simulink model "TST_CrCtl_Governor"  (R2016b)
settings: Solver=FixedStepDiscrete  StartTime=0.0  StopTime=simTime  FixedStep=sampleTime  RelTol=1e-3
values from neighbouring files (symbols this model uses):
  testCase = 1    [initTST_CrCtl_Governor_001.m]    (also in initTST_CrCtl_Governor_002.m = 2; initTST_CrCtl_Governor_003.m = 3; initTST_CrCtl_Governor_004.m = 4; initTST_CrCtl_Governor_005.m = 5)
libraries: simulink x144, UnitTest_Lib x110
(part 3 of 7)

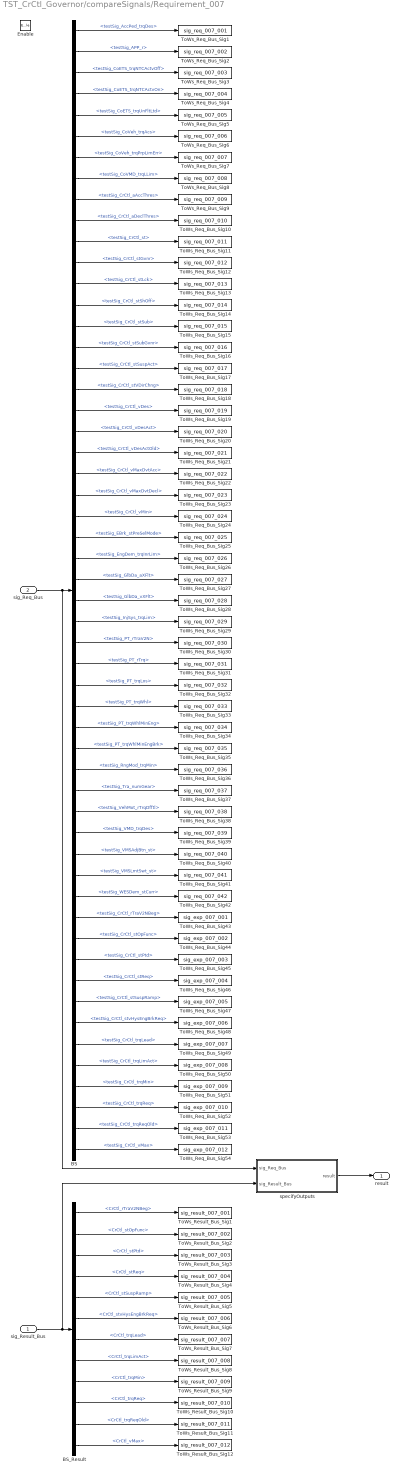
== system TST_CrCtl_Governor/compareSignals/Requirement_007 ==
  sig_Result_Bus : Inport
  sig_Req_Bus : Inport  Port=2
  Enable : EnablePort
  BS : BusSelector  OutputSignals=testSig_AccPed_trqDes,testSig_APP_r,testSig_CoETS_trqNTCActvOff,testSig_CoETS_trqNTCActvOn,testSig_CoETS_trqUnFltLtd,testSig_CoVeh_trqAcs,testSig_CoVeh_trqPrpLimErr,testSig_CoVMD_trqLLim,testSig_CrCtl_aAccThres,testSig_CrCtl_aDeclThres,testSig_CrCtl_st,testSig_CrCtl_stGvnr,testSig_CrCtl_stLck,testSig_CrCtl_stShOff,testSig_CrCtl_stSub,testSig_CrCtl_stSubGvnr,testSig_CrCtl_stSuspAct,testSig_CrCtl_stVDirChng,testSig_CrCtl_vDes,testSig_CrCtl_vDesAct,testSig_CrCtl_vDesActOld,testSig_CrCtl_vMaxDvtAcc,testSig_CrCtl_vMaxDvtDecl,testSig_CrCtl_vMin,testSig_EBrk_stPreSelMode,testSig_EngDem_trqInrLim,testSig_GlbDa_aXFlt,testSig_GlbDa_vXFlt,testSig_InjSys_trqLim,testSig_PT_rTraV2N,testSig_PT_rTrq,testSig_PT_trqLos,testSig_PT_trqWhl,testSig_PT_trqWhlMinEng,testSig_PT_trqWhlMinEngBrk,testSig_RngMod_trqMin,testSig_Tra_numGear,testSig_VehMot_rTrqDfftl,testSig_VMD_trqDes,testSig_VMSAdjBtn_st,testSig_VMSLmtSwt_st,testSig_WESDem_stCurr,testSig_CrCtl_rTraV2NBeg,testSig_CrCtl_stOpFunc,testSig_CrCtl_stPtd,testSig_CrCtl_stReq,testSig_CrCtl_stSuspRamp,testSig_CrCtl_stvHysEngBrkReq,testSig_CrCtl_trqLead,testSig_CrCtl_trqLimAct,testSig_CrCtl_trqMin,testSig_CrCtl_trqReq,testSig_CrCtl_trqReqOld,testSig_CrCtl_vMax
  BS_Result : BusSelector  OutputSignals=CrCtl_rTraV2NBeg,CrCtl_stOpFunc,CrCtl_stPtd,CrCtl_stReq,CrCtl_stSuspRamp,CrCtl_stvHysEngBrkReq,CrCtl_trqLead,CrCtl_trqLimAct,CrCtl_trqMin,CrCtl_trqReq,CrCtl_trqReqOld,CrCtl_vMax
  ToWs_Req_Bus_Sig1 : ToWorkspace  VariableName=sig_req_007_001  SaveFormat=Structure With Time
  ToWs_Req_Bus_Sig10 : ToWorkspace  VariableName=sig_req_007_010  SaveFormat=Structure With Time
  ToWs_Req_Bus_Sig11 : ToWorkspace  VariableName=sig_req_007_011  SaveFormat=Structure With Time
  ToWs_Req_Bus_Sig12 : ToWorkspace  VariableName=sig_req_007_012  SaveFormat=Structure With Time
  ToWs_Req_Bus_Sig13 : ToWorkspace  VariableName=sig_req_007_013  SaveFormat=Structure With Time
  ToWs_Req_Bus_Sig14 : ToWorkspace  VariableName=sig_req_007_014  SaveFormat=Structure With Time
  ToWs_Req_Bus_Sig15 : ToWorkspace  VariableName=sig_req_007_015  SaveFormat=Structure With Time
  ToWs_Req_Bus_Sig16 : ToWorkspace  VariableName=sig_req_007_016  SaveFormat=Structure With Time
  ToWs_Req_Bus_Sig17 : ToWorkspace  VariableName=sig_req_007_017  SaveFormat=Structure With Time
  ToWs_Req_Bus_Sig18 : ToWorkspace  VariableName=sig_req_007_018  SaveFormat=Structure With Time
  ToWs_Req_Bus_Sig19 : ToWorkspace  VariableName=sig_req_007_019  SaveFormat=Structure With Time
  ToWs_Req_Bus_Sig2 : ToWorkspace  VariableName=sig_req_007_002  SaveFormat=Structure With Time
  ToWs_Req_Bus_Sig20 : ToWorkspace  VariableName=sig_req_007_020  SaveFormat=Structure With Time
  ToWs_Req_Bus_Sig21 : ToWorkspace  VariableName=sig_req_007_021  SaveFormat=Structure With Time
  ToWs_Req_Bus_Sig22 : ToWorkspace  VariableName=sig_req_007_022  SaveFormat=Structure With Time
  ToWs_Req_Bus_Sig23 : ToWorkspace  VariableName=sig_req_007_023  SaveFormat=Structure With Time
  ToWs_Req_Bus_Sig24 : ToWorkspace  VariableName=sig_req_007_024  SaveFormat=Structure With Time
  ToWs_Req_Bus_Sig25 : ToWorkspace  VariableName=sig_req_007_025  SaveFormat=Structure With Time
  ToWs_Req_Bus_Sig26 : ToWorkspace  VariableName=sig_req_007_026  SaveFormat=Structure With Time
  ToWs_Req_Bus_Sig27 : ToWorkspace  VariableName=sig_req_007_027  SaveFormat=Structure With Time
  ToWs_Req_Bus_Sig28 : ToWorkspace  VariableName=sig_req_007_028  SaveFormat=Structure With Time
  ToWs_Req_Bus_Sig29 : ToWorkspace  VariableName=sig_req_007_029  SaveFormat=Structure With Time
  ToWs_Req_Bus_Sig3 : ToWorkspace  VariableName=sig_req_007_003  SaveFormat=Structure With Time
  ToWs_Req_Bus_Sig30 : ToWorkspace  VariableName=sig_req_007_030  SaveFormat=Structure With Time
  ToWs_Req_Bus_Sig31 : ToWorkspace  VariableName=sig_req_007_031  SaveFormat=Structure With Time
  ToWs_Req_Bus_Sig32 : ToWorkspace  VariableName=sig_req_007_032  SaveFormat=Structure With Time
  ToWs_Req_Bus_Sig33 : ToWorkspace  VariableName=sig_req_007_033  SaveFormat=Structure With Time
  ToWs_Req_Bus_Sig34 : ToWorkspace  VariableName=sig_req_007_034  SaveFormat=Structure With Time
  ToWs_Req_Bus_Sig35 : ToWorkspace  VariableName=sig_req_007_035  SaveFormat=Structure With Time
  ToWs_Req_Bus_Sig36 : ToWorkspace  VariableName=sig_req_007_036  SaveFormat=Structure With Time
  ToWs_Req_Bus_Sig37 : ToWorkspace  VariableName=sig_req_007_037  SaveFormat=Structure With Time
  ToWs_Req_Bus_Sig38 : ToWorkspace  VariableName=sig_req_007_038  SaveFormat=Structure With Time
  ToWs_Req_Bus_Sig39 : ToWorkspace  VariableName=sig_req_007_039  SaveFormat=Structure With Time
  ToWs_Req_Bus_Sig4 : ToWorkspace  VariableName=sig_req_007_004  SaveFormat=Structure With Time
  ToWs_Req_Bus_Sig40 : ToWorkspace  VariableName=sig_req_007_040  SaveFormat=Structure With Time
  ToWs_Req_Bus_Sig41 : ToWorkspace  VariableName=sig_req_007_041  SaveFormat=Structure With Time
  ToWs_Req_Bus_Sig42 : ToWorkspace  VariableName=sig_req_007_042  SaveFormat=Structure With Time
  ToWs_Req_Bus_Sig43 : ToWorkspace  VariableName=sig_exp_007_001  SaveFormat=Structure With Time
  ToWs_Req_Bus_Sig44 : ToWorkspace  VariableName=sig_exp_007_002  SaveFormat=Structure With Time
  ToWs_Req_Bus_Sig45 : ToWorkspace  VariableName=sig_exp_007_003  SaveFormat=Structure With Time
  ToWs_Req_Bus_Sig46 : ToWorkspace  VariableName=sig_exp_007_004  SaveFormat=Structure With Time
  ToWs_Req_Bus_Sig47 : ToWorkspace  VariableName=sig_exp_007_005  SaveFormat=Structure With Time
  ToWs_Req_Bus_Sig48 : ToWorkspace  VariableName=sig_exp_007_006  SaveFormat=Structure With Time
  ToWs_Req_Bus_Sig49 : ToWorkspace  VariableName=sig_exp_007_007  SaveFormat=Structure With Time
  ToWs_Req_Bus_Sig5 : ToWorkspace  VariableName=sig_req_007_005  SaveFormat=Structure With Time
  ToWs_Req_Bus_Sig50 : ToWorkspace  VariableName=sig_exp_007_008  SaveFormat=Structure With Time
  ToWs_Req_Bus_Sig51 : ToWorkspace  VariableName=sig_exp_007_009  SaveFormat=Structure With Time
  ToWs_Req_Bus_Sig52 : ToWorkspace  VariableName=sig_exp_007_010  SaveFormat=Structure With Time
  ToWs_Req_Bus_Sig53 : ToWorkspace  VariableName=sig_exp_007_011  SaveFormat=Structure With Time
  ToWs_Req_Bus_Sig54 : ToWorkspace  VariableName=sig_exp_007_012  SaveFormat=Structure With Time
  ToWs_Req_Bus_Sig6 : ToWorkspace  VariableName=sig_req_007_006  SaveFormat=Structure With Time
  ToWs_Req_Bus_Sig7 : ToWorkspace  VariableName=sig_req_007_007  SaveFormat=Structure With Time
  ToWs_Req_Bus_Sig8 : ToWorkspace  VariableName=sig_req_007_008  SaveFormat=Structure With Time
  ToWs_Req_Bus_Sig9 : ToWorkspace  VariableName=sig_req_007_009  SaveFormat=Structure With Time
  ToWs_Result_Bus_Sig1 : ToWorkspace  VariableName=sig_result_007_001  SaveFormat=Structure With Time
  ToWs_Result_Bus_Sig10 : ToWorkspace  VariableName=sig_result_007_010  SaveFormat=Structure With Time
  ToWs_Result_Bus_Sig11 : ToWorkspace  VariableName=sig_result_007_011  SaveFormat=Structure With Time
  ToWs_Result_Bus_Sig12 : ToWorkspace  VariableName=sig_result_007_012  SaveFormat=Structure With Time
  ToWs_Result_Bus_Sig2 : ToWorkspace  VariableName=sig_result_007_002  SaveFormat=Structure With Time
  ToWs_Result_Bus_Sig3 : ToWorkspace  VariableName=sig_result_007_003  SaveFormat=Structure With Time
  ToWs_Result_Bus_Sig4 : ToWorkspace  VariableName=sig_result_007_004  SaveFormat=Structure With Time
  ToWs_Result_Bus_Sig5 : ToWorkspace  VariableName=sig_result_007_005  SaveFormat=Structure With Time
  ToWs_Result_Bus_Sig6 : ToWorkspace  VariableName=sig_result_007_006  SaveFormat=Structure With Time
  ToWs_Result_Bus_Sig7 : ToWorkspace  VariableName=sig_result_007_007  SaveFormat=Structure With Time
  ToWs_Result_Bus_Sig8 : ToWorkspace  VariableName=sig_result_007_008  SaveFormat=Structure With Time
  ToWs_Result_Bus_Sig9 : ToWorkspace  VariableName=sig_result_007_009  SaveFormat=Structure With Time
  specifyOutputs : Subsystem
  result : Outport
  wires:
  sig_Req_Bus/1 -> BS/1, specifyOutputs/1(sig_Req_Bus)
  BS/1 -> ToWs_Req_Bus_Sig1/1  "<testSig_AccPed_trqDes>"
  BS/2 -> ToWs_Req_Bus_Sig2/1  "<testSig_APP_r>"
  BS/3 -> ToWs_Req_Bus_Sig3/1  "<testSig_CoETS_trqNTCActvOff>"
  BS/4 -> ToWs_Req_Bus_Sig4/1  "<testSig_CoETS_trqNTCActvOn>"
  BS/5 -> ToWs_Req_Bus_Sig5/1  "<testSig_CoETS_trqUnFltLtd>"
  BS/6 -> ToWs_Req_Bus_Sig6/1  "<testSig_CoVeh_trqAcs>"
  BS/7 -> ToWs_Req_Bus_Sig7/1  "<testSig_CoVeh_trqPrpLimErr>"
  BS/8 -> ToWs_Req_Bus_Sig8/1  "<testSig_CoVMD_trqLLim>"
  BS/9 -> ToWs_Req_Bus_Sig9/1  "<testSig_CrCtl_aAccThres>"
  BS/10 -> ToWs_Req_Bus_Sig10/1  "<testSig_CrCtl_aDeclThres>"
  BS/11 -> ToWs_Req_Bus_Sig11/1  "<testSig_CrCtl_st>"
  BS/12 -> ToWs_Req_Bus_Sig12/1  "<testSig_CrCtl_stGvnr>"
  BS/13 -> ToWs_Req_Bus_Sig13/1  "<testSig_CrCtl_stLck>"
  BS/14 -> ToWs_Req_Bus_Sig14/1  "<testSig_CrCtl_stShOff>"
  BS/15 -> ToWs_Req_Bus_Sig15/1  "<testSig_CrCtl_stSub>"
  BS/16 -> ToWs_Req_Bus_Sig16/1  "<testSig_CrCtl_stSubGvnr>"
  BS/17 -> ToWs_Req_Bus_Sig17/1  "<testSig_CrCtl_stSuspAct>"
  BS/18 -> ToWs_Req_Bus_Sig18/1  "<testSig_CrCtl_stVDirChng>"
  BS/19 -> ToWs_Req_Bus_Sig19/1  "<testSig_CrCtl_vDes>"
  BS/20 -> ToWs_Req_Bus_Sig20/1  "<testSig_CrCtl_vDesAct>"
  BS/21 -> ToWs_Req_Bus_Sig21/1  "<testSig_CrCtl_vDesActOld>"
  BS/22 -> ToWs_Req_Bus_Sig22/1  "<testSig_CrCtl_vMaxDvtAcc>"
  BS/23 -> ToWs_Req_Bus_Sig23/1  "<testSig_CrCtl_vMaxDvtDecl>"
  BS/24 -> ToWs_Req_Bus_Sig24/1  "<testSig_CrCtl_vMin>"
  BS/25 -> ToWs_Req_Bus_Sig25/1  "<testSig_EBrk_stPreSelMode>"
  BS/26 -> ToWs_Req_Bus_Sig26/1  "<testSig_EngDem_trqInrLim>"
  BS/27 -> ToWs_Req_Bus_Sig27/1  "<testSig_GlbDa_aXFlt>"
  BS/28 -> ToWs_Req_Bus_Sig28/1  "<testSig_GlbDa_vXFlt>"
  BS/29 -> ToWs_Req_Bus_Sig29/1  "<testSig_InjSys_trqLim>"
  BS/30 -> ToWs_Req_Bus_Sig30/1  "<testSig_PT_rTraV2N>"
  BS/31 -> ToWs_Req_Bus_Sig31/1  "<testSig_PT_rTrq>"
  BS/32 -> ToWs_Req_Bus_Sig32/1  "<testSig_PT_trqLos>"
  BS/33 -> ToWs_Req_Bus_Sig33/1  "<testSig_PT_trqWhl>"
  BS/34 -> ToWs_Req_Bus_Sig34/1  "<testSig_PT_trqWhlMinEng>"
  BS/35 -> ToWs_Req_Bus_Sig35/1  "<testSig_PT_trqWhlMinEngBrk>"
  BS/36 -> ToWs_Req_Bus_Sig36/1  "<testSig_RngMod_trqMin>"
  BS/37 -> ToWs_Req_Bus_Sig37/1  "<testSig_Tra_numGear>"
  BS/38 -> ToWs_Req_Bus_Sig38/1  "<testSig_VehMot_rTrqDfftl>"
  BS/39 -> ToWs_Req_Bus_Sig39/1  "<testSig_VMD_trqDes>"
  BS/40 -> ToWs_Req_Bus_Sig40/1  "<testSig_VMSAdjBtn_st>"
  BS/41 -> ToWs_Req_Bus_Sig41/1  "<testSig_VMSLmtSwt_st>"
  BS/42 -> ToWs_Req_Bus_Sig42/1  "<testSig_WESDem_stCurr>"
  BS/43 -> ToWs_Req_Bus_Sig43/1  "<testSig_CrCtl_rTraV2NBeg>"
  BS/44 -> ToWs_Req_Bus_Sig44/1  "<testSig_CrCtl_stOpFunc>"
  BS/45 -> ToWs_Req_Bus_Sig45/1  "<testSig_CrCtl_stPtd>"
  BS/46 -> ToWs_Req_Bus_Sig46/1  "<testSig_CrCtl_stReq>"
  BS/47 -> ToWs_Req_Bus_Sig47/1  "<testSig_CrCtl_stSuspRamp>"
  BS/48 -> ToWs_Req_Bus_Sig48/1  "<testSig_CrCtl_stvHysEngBrkReq>"
  BS/49 -> ToWs_Req_Bus_Sig49/1  "<testSig_CrCtl_trqLead>"
  BS/50 -> ToWs_Req_Bus_Sig50/1  "<testSig_CrCtl_trqLimAct>"
  BS/51 -> ToWs_Req_Bus_Sig51/1  "<testSig_CrCtl_trqMin>"
  BS/52 -> ToWs_Req_Bus_Sig52/1  "<testSig_CrCtl_trqReq>"
  BS/53 -> ToWs_Req_Bus_Sig53/1  "<testSig_CrCtl_trqReqOld>"
  BS/54 -> ToWs_Req_Bus_Sig54/1  "<testSig_CrCtl_vMax>"
  sig_Result_Bus/1 -> BS_Result/1, specifyOutputs/2(sig_Result_Bus)
  BS_Result/1 -> ToWs_Result_Bus_Sig1/1  "<CrCtl_rTraV2NBeg>"
  BS_Result/2 -> ToWs_Result_Bus_Sig2/1  "<CrCtl_stOpFunc>"
  BS_Result/3 -> ToWs_Result_Bus_Sig3/1  "<CrCtl_stPtd>"
  BS_Result/4 -> ToWs_Result_Bus_Sig4/1  "<CrCtl_stReq>"
  BS_Result/5 -> ToWs_Result_Bus_Sig5/1  "<CrCtl_stSuspRamp>"
  BS_Result/6 -> ToWs_Result_Bus_Sig6/1  "<CrCtl_stvHysEngBrkReq>"
  BS_Result/7 -> ToWs_Result_Bus_Sig7/1  "<CrCtl_trqLead>"
  BS_Result/8 -> ToWs_Result_Bus_Sig8/1  "<CrCtl_trqLimAct>"
  BS_Result/9 -> ToWs_Result_Bus_Sig9/1  "<CrCtl_trqMin>"
  BS_Result/10 -> ToWs_Result_Bus_Sig10/1  "<CrCtl_trqReq>"
  BS_Result/11 -> ToWs_Result_Bus_Sig11/1  "<CrCtl_trqReqOld>"
  BS_Result/12 -> ToWs_Result_Bus_Sig12/1  "<CrCtl_vMax>"
  specifyOutputs/1(result) -> result/1

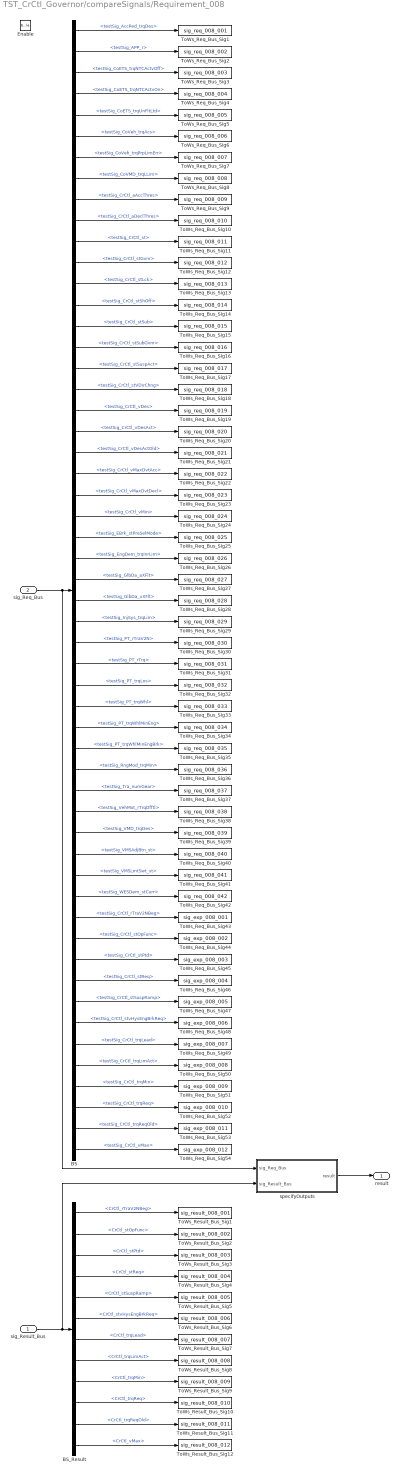
== system TST_CrCtl_Governor/compareSignals/Requirement_008 ==
  sig_Result_Bus : Inport
  sig_Req_Bus : Inport  Port=2
  Enable : EnablePort
  BS : BusSelector  OutputSignals=testSig_AccPed_trqDes,testSig_APP_r,testSig_CoETS_trqNTCActvOff,testSig_CoETS_trqNTCActvOn,testSig_CoETS_trqUnFltLtd,testSig_CoVeh_trqAcs,testSig_CoVeh_trqPrpLimErr,testSig_CoVMD_trqLLim,testSig_CrCtl_aAccThres,testSig_CrCtl_aDeclThres,testSig_CrCtl_st,testSig_CrCtl_stGvnr,testSig_CrCtl_stLck,testSig_CrCtl_stShOff,testSig_CrCtl_stSub,testSig_CrCtl_stSubGvnr,testSig_CrCtl_stSuspAct,testSig_CrCtl_stVDirChng,testSig_CrCtl_vDes,testSig_CrCtl_vDesAct,testSig_CrCtl_vDesActOld,testSig_CrCtl_vMaxDvtAcc,testSig_CrCtl_vMaxDvtDecl,testSig_CrCtl_vMin,testSig_EBrk_stPreSelMode,testSig_EngDem_trqInrLim,testSig_GlbDa_aXFlt,testSig_GlbDa_vXFlt,testSig_InjSys_trqLim,testSig_PT_rTraV2N,testSig_PT_rTrq,testSig_PT_trqLos,testSig_PT_trqWhl,testSig_PT_trqWhlMinEng,testSig_PT_trqWhlMinEngBrk,testSig_RngMod_trqMin,testSig_Tra_numGear,testSig_VehMot_rTrqDfftl,testSig_VMD_trqDes,testSig_VMSAdjBtn_st,testSig_VMSLmtSwt_st,testSig_WESDem_stCurr,testSig_CrCtl_rTraV2NBeg,testSig_CrCtl_stOpFunc,testSig_CrCtl_stPtd,testSig_CrCtl_stReq,testSig_CrCtl_stSuspRamp,testSig_CrCtl_stvHysEngBrkReq,testSig_CrCtl_trqLead,testSig_CrCtl_trqLimAct,testSig_CrCtl_trqMin,testSig_CrCtl_trqReq,testSig_CrCtl_trqReqOld,testSig_CrCtl_vMax
  BS_Result : BusSelector  OutputSignals=CrCtl_rTraV2NBeg,CrCtl_stOpFunc,CrCtl_stPtd,CrCtl_stReq,CrCtl_stSuspRamp,CrCtl_stvHysEngBrkReq,CrCtl_trqLead,CrCtl_trqLimAct,CrCtl_trqMin,CrCtl_trqReq,CrCtl_trqReqOld,CrCtl_vMax
  ToWs_Req_Bus_Sig1 : ToWorkspace  VariableName=sig_req_008_001  SaveFormat=Structure With Time
  ToWs_Req_Bus_Sig10 : ToWorkspace  VariableName=sig_req_008_010  SaveFormat=Structure With Time
  ToWs_Req_Bus_Sig11 : ToWorkspace  VariableName=sig_req_008_011  SaveFormat=Structure With Time
  ToWs_Req_Bus_Sig12 : ToWorkspace  VariableName=sig_req_008_012  SaveFormat=Structure With Time
  ToWs_Req_Bus_Sig13 : ToWorkspace  VariableName=sig_req_008_013  SaveFormat=Structure With Time
  ToWs_Req_Bus_Sig14 : ToWorkspace  VariableName=sig_req_008_014  SaveFormat=Structure With Time
  ToWs_Req_Bus_Sig15 : ToWorkspace  VariableName=sig_req_008_015  SaveFormat=Structure With Time
  ToWs_Req_Bus_Sig16 : ToWorkspace  VariableName=sig_req_008_016  SaveFormat=Structure With Time
  ToWs_Req_Bus_Sig17 : ToWorkspace  VariableName=sig_req_008_017  SaveFormat=Structure With Time
  ToWs_Req_Bus_Sig18 : ToWorkspace  VariableName=sig_req_008_018  SaveFormat=Structure With Time
  ToWs_Req_Bus_Sig19 : ToWorkspace  VariableName=sig_req_008_019  SaveFormat=Structure With Time
  ToWs_Req_Bus_Sig2 : ToWorkspace  VariableName=sig_req_008_002  SaveFormat=Structure With Time
  ToWs_Req_Bus_Sig20 : ToWorkspace  VariableName=sig_req_008_020  SaveFormat=Structure With Time
  ToWs_Req_Bus_Sig21 : ToWorkspace  VariableName=sig_req_008_021  SaveFormat=Structure With Time
  ToWs_Req_Bus_Sig22 : ToWorkspace  VariableName=sig_req_008_022  SaveFormat=Structure With Time
  ToWs_Req_Bus_Sig23 : ToWorkspace  VariableName=sig_req_008_023  SaveFormat=Structure With Time
  ToWs_Req_Bus_Sig24 : ToWorkspace  VariableName=sig_req_008_024  SaveFormat=Structure With Time
  ToWs_Req_Bus_Sig25 : ToWorkspace  VariableName=sig_req_008_025  SaveFormat=Structure With Time
  ToWs_Req_Bus_Sig26 : ToWorkspace  VariableName=sig_req_008_026  SaveFormat=Structure With Time
  ToWs_Req_Bus_Sig27 : ToWorkspace  VariableName=sig_req_008_027  SaveFormat=Structure With Time
  ToWs_Req_Bus_Sig28 : ToWorkspace  VariableName=sig_req_008_028  SaveFormat=Structure With Time
  ToWs_Req_Bus_Sig29 : ToWorkspace  VariableName=sig_req_008_029  SaveFormat=Structure With Time
  ToWs_Req_Bus_Sig3 : ToWorkspace  VariableName=sig_req_008_003  SaveFormat=Structure With Time
  ToWs_Req_Bus_Sig30 : ToWorkspace  VariableName=sig_req_008_030  SaveFormat=Structure With Time
  ToWs_Req_Bus_Sig31 : ToWorkspace  VariableName=sig_req_008_031  SaveFormat=Structure With Time
  ToWs_Req_Bus_Sig32 : ToWorkspace  VariableName=sig_req_008_032  SaveFormat=Structure With Time
  ToWs_Req_Bus_Sig33 : ToWorkspace  VariableName=sig_req_008_033  SaveFormat=Structure With Time
  ToWs_Req_Bus_Sig34 : ToWorkspace  VariableName=sig_req_008_034  SaveFormat=Structure With Time
  ToWs_Req_Bus_Sig35 : ToWorkspace  VariableName=sig_req_008_035  SaveFormat=Structure With Time
  ToWs_Req_Bus_Sig36 : ToWorkspace  VariableName=sig_req_008_036  SaveFormat=Structure With Time
  ToWs_Req_Bus_Sig37 : ToWorkspace  VariableName=sig_req_008_037  SaveFormat=Structure With Time
  ToWs_Req_Bus_Sig38 : ToWorkspace  VariableName=sig_req_008_038  SaveFormat=Structure With Time
  ToWs_Req_Bus_Sig39 : ToWorkspace  VariableName=sig_req_008_039  SaveFormat=Structure With Time
  ToWs_Req_Bus_Sig4 : ToWorkspace  VariableName=sig_req_008_004  SaveFormat=Structure With Time
  ToWs_Req_Bus_Sig40 : ToWorkspace  VariableName=sig_req_008_040  SaveFormat=Structure With Time
  ToWs_Req_Bus_Sig41 : ToWorkspace  VariableName=sig_req_008_041  SaveFormat=Structure With Time
  ToWs_Req_Bus_Sig42 : ToWorkspace  VariableName=sig_req_008_042  SaveFormat=Structure With Time
  ToWs_Req_Bus_Sig43 : ToWorkspace  VariableName=sig_exp_008_001  SaveFormat=Structure With Time
  ToWs_Req_Bus_Sig44 : ToWorkspace  VariableName=sig_exp_008_002  SaveFormat=Structure With Time
  ToWs_Req_Bus_Sig45 : ToWorkspace  VariableName=sig_exp_008_003  SaveFormat=Structure With Time
  ToWs_Req_Bus_Sig46 : ToWorkspace  VariableName=sig_exp_008_004  SaveFormat=Structure With Time
  ToWs_Req_Bus_Sig47 : ToWorkspace  VariableName=sig_exp_008_005  SaveFormat=Structure With Time
  ToWs_Req_Bus_Sig48 : ToWorkspace  VariableName=sig_exp_008_006  SaveFormat=Structure With Time
  ToWs_Req_Bus_Sig49 : ToWorkspace  VariableName=sig_exp_008_007  SaveFormat=Structure With Time
  ToWs_Req_Bus_Sig5 : ToWorkspace  VariableName=sig_req_008_005  SaveFormat=Structure With Time
  ToWs_Req_Bus_Sig50 : ToWorkspace  VariableName=sig_exp_008_008  SaveFormat=Structure With Time
  ToWs_Req_Bus_Sig51 : ToWorkspace  VariableName=sig_exp_008_009  SaveFormat=Structure With Time
  ToWs_Req_Bus_Sig52 : ToWorkspace  VariableName=sig_exp_008_010  SaveFormat=Structure With Time
  ToWs_Req_Bus_Sig53 : ToWorkspace  VariableName=sig_exp_008_011  SaveFormat=Structure With Time
  ToWs_Req_Bus_Sig54 : ToWorkspace  VariableName=sig_exp_008_012  SaveFormat=Structure With Time
  ToWs_Req_Bus_Sig6 : ToWorkspace  VariableName=sig_req_008_006  SaveFormat=Structure With Time
  ToWs_Req_Bus_Sig7 : ToWorkspace  VariableName=sig_req_008_007  SaveFormat=Structure With Time
  ToWs_Req_Bus_Sig8 : ToWorkspace  VariableName=sig_req_008_008  SaveFormat=Structure With Time
  ToWs_Req_Bus_Sig9 : ToWorkspace  VariableName=sig_req_008_009  SaveFormat=Structure With Time
  ToWs_Result_Bus_Sig1 : ToWorkspace  VariableName=sig_result_008_001  SaveFormat=Structure With Time
  ToWs_Result_Bus_Sig10 : ToWorkspace  VariableName=sig_result_008_010  SaveFormat=Structure With Time
  ToWs_Result_Bus_Sig11 : ToWorkspace  VariableName=sig_result_008_011  SaveFormat=Structure With Time
  ToWs_Result_Bus_Sig12 : ToWorkspace  VariableName=sig_result_008_012  SaveFormat=Structure With Time
  ToWs_Result_Bus_Sig2 : ToWorkspace  VariableName=sig_result_008_002  SaveFormat=Structure With Time
  ToWs_Result_Bus_Sig3 : ToWorkspace  VariableName=sig_result_008_003  SaveFormat=Structure With Time
  ToWs_Result_Bus_Sig4 : ToWorkspace  VariableName=sig_result_008_004  SaveFormat=Structure With Time
  ToWs_Result_Bus_Sig5 : ToWorkspace  VariableName=sig_result_008_005  SaveFormat=Structure With Time
  ToWs_Result_Bus_Sig6 : ToWorkspace  VariableName=sig_result_008_006  SaveFormat=Structure With Time
  ToWs_Result_Bus_Sig7 : ToWorkspace  VariableName=sig_result_008_007  SaveFormat=Structure With Time
  ToWs_Result_Bus_Sig8 : ToWorkspace  VariableName=sig_result_008_008  SaveFormat=Structure With Time
  ToWs_Result_Bus_Sig9 : ToWorkspace  VariableName=sig_result_008_009  SaveFormat=Structure With Time
  specifyOutputs : Subsystem
  result : Outport
  wires:
  sig_Req_Bus/1 -> BS/1, specifyOutputs/1(sig_Req_Bus)
  BS/1 -> ToWs_Req_Bus_Sig1/1  "<testSig_AccPed_trqDes>"
  BS/2 -> ToWs_Req_Bus_Sig2/1  "<testSig_APP_r>"
  BS/3 -> ToWs_Req_Bus_Sig3/1  "<testSig_CoETS_trqNTCActvOff>"
  BS/4 -> ToWs_Req_Bus_Sig4/1  "<testSig_CoETS_trqNTCActvOn>"
  BS/5 -> ToWs_Req_Bus_Sig5/1  "<testSig_CoETS_trqUnFltLtd>"
  BS/6 -> ToWs_Req_Bus_Sig6/1  "<testSig_CoVeh_trqAcs>"
  BS/7 -> ToWs_Req_Bus_Sig7/1  "<testSig_CoVeh_trqPrpLimErr>"
  BS/8 -> ToWs_Req_Bus_Sig8/1  "<testSig_CoVMD_trqLLim>"
  BS/9 -> ToWs_Req_Bus_Sig9/1  "<testSig_CrCtl_aAccThres>"
  BS/10 -> ToWs_Req_Bus_Sig10/1  "<testSig_CrCtl_aDeclThres>"
  BS/11 -> ToWs_Req_Bus_Sig11/1  "<testSig_CrCtl_st>"
  BS/12 -> ToWs_Req_Bus_Sig12/1  "<testSig_CrCtl_stGvnr>"
  BS/13 -> ToWs_Req_Bus_Sig13/1  "<testSig_CrCtl_stLck>"
  BS/14 -> ToWs_Req_Bus_Sig14/1  "<testSig_CrCtl_stShOff>"
  BS/15 -> ToWs_Req_Bus_Sig15/1  "<testSig_CrCtl_stSub>"
  BS/16 -> ToWs_Req_Bus_Sig16/1  "<testSig_CrCtl_stSubGvnr>"
  BS/17 -> ToWs_Req_Bus_Sig17/1  "<testSig_CrCtl_stSuspAct>"
  BS/18 -> ToWs_Req_Bus_Sig18/1  "<testSig_CrCtl_stVDirChng>"
  BS/19 -> ToWs_Req_Bus_Sig19/1  "<testSig_CrCtl_vDes>"
  BS/20 -> ToWs_Req_Bus_Sig20/1  "<testSig_CrCtl_vDesAct>"
  BS/21 -> ToWs_Req_Bus_Sig21/1  "<testSig_CrCtl_vDesActOld>"
  BS/22 -> ToWs_Req_Bus_Sig22/1  "<testSig_CrCtl_vMaxDvtAcc>"
  BS/23 -> ToWs_Req_Bus_Sig23/1  "<testSig_CrCtl_vMaxDvtDecl>"
  BS/24 -> ToWs_Req_Bus_Sig24/1  "<testSig_CrCtl_vMin>"
  BS/25 -> ToWs_Req_Bus_Sig25/1  "<testSig_EBrk_stPreSelMode>"
  BS/26 -> ToWs_Req_Bus_Sig26/1  "<testSig_EngDem_trqInrLim>"
  BS/27 -> ToWs_Req_Bus_Sig27/1  "<testSig_GlbDa_aXFlt>"
  BS/28 -> ToWs_Req_Bus_Sig28/1  "<testSig_GlbDa_vXFlt>"
  BS/29 -> ToWs_Req_Bus_Sig29/1  "<testSig_InjSys_trqLim>"
  BS/30 -> ToWs_Req_Bus_Sig30/1  "<testSig_PT_rTraV2N>"
  BS/31 -> ToWs_Req_Bus_Sig31/1  "<testSig_PT_rTrq>"
  BS/32 -> ToWs_Req_Bus_Sig32/1  "<testSig_PT_trqLos>"
  BS/33 -> ToWs_Req_Bus_Sig33/1  "<testSig_PT_trqWhl>"
  BS/34 -> ToWs_Req_Bus_Sig34/1  "<testSig_PT_trqWhlMinEng>"
  BS/35 -> ToWs_Req_Bus_Sig35/1  "<testSig_PT_trqWhlMinEngBrk>"
  BS/36 -> ToWs_Req_Bus_Sig36/1  "<testSig_RngMod_trqMin>"
  BS/37 -> ToWs_Req_Bus_Sig37/1  "<testSig_Tra_numGear>"
  BS/38 -> ToWs_Req_Bus_Sig38/1  "<testSig_VehMot_rTrqDfftl>"
  BS/39 -> ToWs_Req_Bus_Sig39/1  "<testSig_VMD_trqDes>"
  BS/40 -> ToWs_Req_Bus_Sig40/1  "<testSig_VMSAdjBtn_st>"
  BS/41 -> ToWs_Req_Bus_Sig41/1  "<testSig_VMSLmtSwt_st>"
  BS/42 -> ToWs_Req_Bus_Sig42/1  "<testSig_WESDem_stCurr>"
  BS/43 -> ToWs_Req_Bus_Sig43/1  "<testSig_CrCtl_rTraV2NBeg>"
  BS/44 -> ToWs_Req_Bus_Sig44/1  "<testSig_CrCtl_stOpFunc>"
  BS/45 -> ToWs_Req_Bus_Sig45/1  "<testSig_CrCtl_stPtd>"
  BS/46 -> ToWs_Req_Bus_Sig46/1  "<testSig_CrCtl_stReq>"
  BS/47 -> ToWs_Req_Bus_Sig47/1  "<testSig_CrCtl_stSuspRamp>"
  BS/48 -> ToWs_Req_Bus_Sig48/1  "<testSig_CrCtl_stvHysEngBrkReq>"
  BS/49 -> ToWs_Req_Bus_Sig49/1  "<testSig_CrCtl_trqLead>"
  BS/50 -> ToWs_Req_Bus_Sig50/1  "<testSig_CrCtl_trqLimAct>"
  BS/51 -> ToWs_Req_Bus_Sig51/1  "<testSig_CrCtl_trqMin>"
  BS/52 -> ToWs_Req_Bus_Sig52/1  "<testSig_CrCtl_trqReq>"
  BS/53 -> ToWs_Req_Bus_Sig53/1  "<testSig_CrCtl_trqReqOld>"
  BS/54 -> ToWs_Req_Bus_Sig54/1  "<testSig_CrCtl_vMax>"
  sig_Result_Bus/1 -> BS_Result/1, specifyOutputs/2(sig_Result_Bus)
  BS_Result/1 -> ToWs_Result_Bus_Sig1/1  "<CrCtl_rTraV2NBeg>"
  BS_Result/2 -> ToWs_Result_Bus_Sig2/1  "<CrCtl_stOpFunc>"
  BS_Result/3 -> ToWs_Result_Bus_Sig3/1  "<CrCtl_stPtd>"
  BS_Result/4 -> ToWs_Result_Bus_Sig4/1  "<CrCtl_stReq>"
  BS_Result/5 -> ToWs_Result_Bus_Sig5/1  "<CrCtl_stSuspRamp>"
  BS_Result/6 -> ToWs_Result_Bus_Sig6/1  "<CrCtl_stvHysEngBrkReq>"
  BS_Result/7 -> ToWs_Result_Bus_Sig7/1  "<CrCtl_trqLead>"
  BS_Result/8 -> ToWs_Result_Bus_Sig8/1  "<CrCtl_trqLimAct>"
  BS_Result/9 -> ToWs_Result_Bus_Sig9/1  "<CrCtl_trqMin>"
  BS_Result/10 -> ToWs_Result_Bus_Sig10/1  "<CrCtl_trqReq>"
  BS_Result/11 -> ToWs_Result_Bus_Sig11/1  "<CrCtl_trqReqOld>"
  BS_Result/12 -> ToWs_Result_Bus_Sig12/1  "<CrCtl_vMax>"
  specifyOutputs/1(result) -> result/1

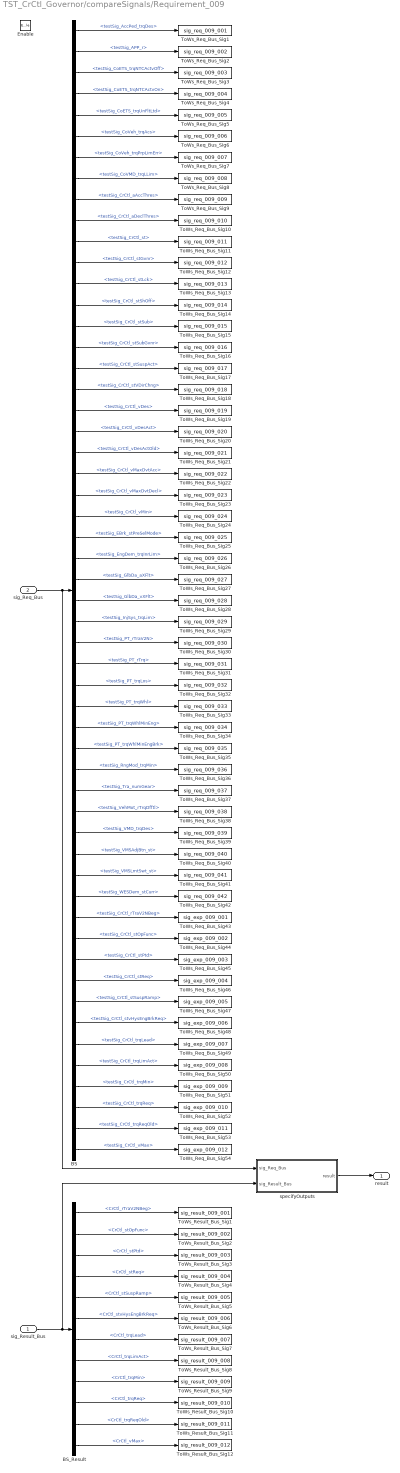
== system TST_CrCtl_Governor/compareSignals/Requirement_009 ==
  sig_Result_Bus : Inport
  sig_Req_Bus : Inport  Port=2
  Enable : EnablePort
  BS : BusSelector  OutputSignals=testSig_AccPed_trqDes,testSig_APP_r,testSig_CoETS_trqNTCActvOff,testSig_CoETS_trqNTCActvOn,testSig_CoETS_trqUnFltLtd,testSig_CoVeh_trqAcs,testSig_CoVeh_trqPrpLimErr,testSig_CoVMD_trqLLim,testSig_CrCtl_aAccThres,testSig_CrCtl_aDeclThres,testSig_CrCtl_st,testSig_CrCtl_stGvnr,testSig_CrCtl_stLck,testSig_CrCtl_stShOff,testSig_CrCtl_stSub,testSig_CrCtl_stSubGvnr,testSig_CrCtl_stSuspAct,testSig_CrCtl_stVDirChng,testSig_CrCtl_vDes,testSig_CrCtl_vDesAct,testSig_CrCtl_vDesActOld,testSig_CrCtl_vMaxDvtAcc,testSig_CrCtl_vMaxDvtDecl,testSig_CrCtl_vMin,testSig_EBrk_stPreSelMode,testSig_EngDem_trqInrLim,testSig_GlbDa_aXFlt,testSig_GlbDa_vXFlt,testSig_InjSys_trqLim,testSig_PT_rTraV2N,testSig_PT_rTrq,testSig_PT_trqLos,testSig_PT_trqWhl,testSig_PT_trqWhlMinEng,testSig_PT_trqWhlMinEngBrk,testSig_RngMod_trqMin,testSig_Tra_numGear,testSig_VehMot_rTrqDfftl,testSig_VMD_trqDes,testSig_VMSAdjBtn_st,testSig_VMSLmtSwt_st,testSig_WESDem_stCurr,testSig_CrCtl_rTraV2NBeg,testSig_CrCtl_stOpFunc,testSig_CrCtl_stPtd,testSig_CrCtl_stReq,testSig_CrCtl_stSuspRamp,testSig_CrCtl_stvHysEngBrkReq,testSig_CrCtl_trqLead,testSig_CrCtl_trqLimAct,testSig_CrCtl_trqMin,testSig_CrCtl_trqReq,testSig_CrCtl_trqReqOld,testSig_CrCtl_vMax
  BS_Result : BusSelector  OutputSignals=CrCtl_rTraV2NBeg,CrCtl_stOpFunc,CrCtl_stPtd,CrCtl_stReq,CrCtl_stSuspRamp,CrCtl_stvHysEngBrkReq,CrCtl_trqLead,CrCtl_trqLimAct,CrCtl_trqMin,CrCtl_trqReq,CrCtl_trqReqOld,CrCtl_vMax
  ToWs_Req_Bus_Sig1 : ToWorkspace  VariableName=sig_req_009_001  SaveFormat=Structure With Time
  ToWs_Req_Bus_Sig10 : ToWorkspace  VariableName=sig_req_009_010  SaveFormat=Structure With Time
  ToWs_Req_Bus_Sig11 : ToWorkspace  VariableName=sig_req_009_011  SaveFormat=Structure With Time
  ToWs_Req_Bus_Sig12 : ToWorkspace  VariableName=sig_req_009_012  SaveFormat=Structure With Time
  ToWs_Req_Bus_Sig13 : ToWorkspace  VariableName=sig_req_009_013  SaveFormat=Structure With Time
  ToWs_Req_Bus_Sig14 : ToWorkspace  VariableName=sig_req_009_014  SaveFormat=Structure With Time
  ToWs_Req_Bus_Sig15 : ToWorkspace  VariableName=sig_req_009_015  SaveFormat=Structure With Time
  ToWs_Req_Bus_Sig16 : ToWorkspace  VariableName=sig_req_009_016  SaveFormat=Structure With Time
  ToWs_Req_Bus_Sig17 : ToWorkspace  VariableName=sig_req_009_017  SaveFormat=Structure With Time
  ToWs_Req_Bus_Sig18 : ToWorkspace  VariableName=sig_req_009_018  SaveFormat=Structure With Time
  ToWs_Req_Bus_Sig19 : ToWorkspace  VariableName=sig_req_009_019  SaveFormat=Structure With Time
  ToWs_Req_Bus_Sig2 : ToWorkspace  VariableName=sig_req_009_002  SaveFormat=Structure With Time
  ToWs_Req_Bus_Sig20 : ToWorkspace  VariableName=sig_req_009_020  SaveFormat=Structure With Time
  ToWs_Req_Bus_Sig21 : ToWorkspace  VariableName=sig_req_009_021  SaveFormat=Structure With Time
  ToWs_Req_Bus_Sig22 : ToWorkspace  VariableName=sig_req_009_022  SaveFormat=Structure With Time
  ToWs_Req_Bus_Sig23 : ToWorkspace  VariableName=sig_req_009_023  SaveFormat=Structure With Time
  ToWs_Req_Bus_Sig24 : ToWorkspace  VariableName=sig_req_009_024  SaveFormat=Structure With Time
  ToWs_Req_Bus_Sig25 : ToWorkspace  VariableName=sig_req_009_025  SaveFormat=Structure With Time
  ToWs_Req_Bus_Sig26 : ToWorkspace  VariableName=sig_req_009_026  SaveFormat=Structure With Time
  ToWs_Req_Bus_Sig27 : ToWorkspace  VariableName=sig_req_009_027  SaveFormat=Structure With Time
  ToWs_Req_Bus_Sig28 : ToWorkspace  VariableName=sig_req_009_028  SaveFormat=Structure With Time
  ToWs_Req_Bus_Sig29 : ToWorkspace  VariableName=sig_req_009_029  SaveFormat=Structure With Time
  ToWs_Req_Bus_Sig3 : ToWorkspace  VariableName=sig_req_009_003  SaveFormat=Structure With Time
  ToWs_Req_Bus_Sig30 : ToWorkspace  VariableName=sig_req_009_030  SaveFormat=Structure With Time
  ToWs_Req_Bus_Sig31 : ToWorkspace  VariableName=sig_req_009_031  SaveFormat=Structure With Time
  ToWs_Req_Bus_Sig32 : ToWorkspace  VariableName=sig_req_009_032  SaveFormat=Structure With Time
  ToWs_Req_Bus_Sig33 : ToWorkspace  VariableName=sig_req_009_033  SaveFormat=Structure With Time
  ToWs_Req_Bus_Sig34 : ToWorkspace  VariableName=sig_req_009_034  SaveFormat=Structure With Time
  ToWs_Req_Bus_Sig35 : ToWorkspace  VariableName=sig_req_009_035  SaveFormat=Structure With Time
  ToWs_Req_Bus_Sig36 : ToWorkspace  VariableName=sig_req_009_036  SaveFormat=Structure With Time
  ToWs_Req_Bus_Sig37 : ToWorkspace  VariableName=sig_req_009_037  SaveFormat=Structure With Time
  ToWs_Req_Bus_Sig38 : ToWorkspace  VariableName=sig_req_009_038  SaveFormat=Structure With Time
  ToWs_Req_Bus_Sig39 : ToWorkspace  VariableName=sig_req_009_039  SaveFormat=Structure With Time
  ToWs_Req_Bus_Sig4 : ToWorkspace  VariableName=sig_req_009_004  SaveFormat=Structure With Time
  ToWs_Req_Bus_Sig40 : ToWorkspace  VariableName=sig_req_009_040  SaveFormat=Structure With Time
  ToWs_Req_Bus_Sig41 : ToWorkspace  VariableName=sig_req_009_041  SaveFormat=Structure With Time
  ToWs_Req_Bus_Sig42 : ToWorkspace  VariableName=sig_req_009_042  SaveFormat=Structure With Time
  ToWs_Req_Bus_Sig43 : ToWorkspace  VariableName=sig_exp_009_001  SaveFormat=Structure With Time
  ToWs_Req_Bus_Sig44 : ToWorkspace  VariableName=sig_exp_009_002  SaveFormat=Structure With Time
  ToWs_Req_Bus_Sig45 : ToWorkspace  VariableName=sig_exp_009_003  SaveFormat=Structure With Time
  ToWs_Req_Bus_Sig46 : ToWorkspace  VariableName=sig_exp_009_004  SaveFormat=Structure With Time
  ToWs_Req_Bus_Sig47 : ToWorkspace  VariableName=sig_exp_009_005  SaveFormat=Structure With Time
  ToWs_Req_Bus_Sig48 : ToWorkspace  VariableName=sig_exp_009_006  SaveFormat=Structure With Time
  ToWs_Req_Bus_Sig49 : ToWorkspace  VariableName=sig_exp_009_007  SaveFormat=Structure With Time
  ToWs_Req_Bus_Sig5 : ToWorkspace  VariableName=sig_req_009_005  SaveFormat=Structure With Time
  ToWs_Req_Bus_Sig50 : ToWorkspace  VariableName=sig_exp_009_008  SaveFormat=Structure With Time
  ToWs_Req_Bus_Sig51 : ToWorkspace  VariableName=sig_exp_009_009  SaveFormat=Structure With Time
  ToWs_Req_Bus_Sig52 : ToWorkspace  VariableName=sig_exp_009_010  SaveFormat=Structure With Time
  ToWs_Req_Bus_Sig53 : ToWorkspace  VariableName=sig_exp_009_011  SaveFormat=Structure With Time
  ToWs_Req_Bus_Sig54 : ToWorkspace  VariableName=sig_exp_009_012  SaveFormat=Structure With Time
  ToWs_Req_Bus_Sig6 : ToWorkspace  VariableName=sig_req_009_006  SaveFormat=Structure With Time
  ToWs_Req_Bus_Sig7 : ToWorkspace  VariableName=sig_req_009_007  SaveFormat=Structure With Time
  ToWs_Req_Bus_Sig8 : ToWorkspace  VariableName=sig_req_009_008  SaveFormat=Structure With Time
  ToWs_Req_Bus_Sig9 : ToWorkspace  VariableName=sig_req_009_009  SaveFormat=Structure With Time
  ToWs_Result_Bus_Sig1 : ToWorkspace  VariableName=sig_result_009_001  SaveFormat=Structure With Time
  ToWs_Result_Bus_Sig10 : ToWorkspace  VariableName=sig_result_009_010  SaveFormat=Structure With Time
  ToWs_Result_Bus_Sig11 : ToWorkspace  VariableName=sig_result_009_011  SaveFormat=Structure With Time
  ToWs_Result_Bus_Sig12 : ToWorkspace  VariableName=sig_result_009_012  SaveFormat=Structure With Time
  ToWs_Result_Bus_Sig2 : ToWorkspace  VariableName=sig_result_009_002  SaveFormat=Structure With Time
  ToWs_Result_Bus_Sig3 : ToWorkspace  VariableName=sig_result_009_003  SaveFormat=Structure With Time
  ToWs_Result_Bus_Sig4 : ToWorkspace  VariableName=sig_result_009_004  SaveFormat=Structure With Time
  ToWs_Result_Bus_Sig5 : ToWorkspace  VariableName=sig_result_009_005  SaveFormat=Structure With Time
  ToWs_Result_Bus_Sig6 : ToWorkspace  VariableName=sig_result_009_006  SaveFormat=Structure With Time
  ToWs_Result_Bus_Sig7 : ToWorkspace  VariableName=sig_result_009_007  SaveFormat=Structure With Time
  ToWs_Result_Bus_Sig8 : ToWorkspace  VariableName=sig_result_009_008  SaveFormat=Structure With Time
  ToWs_Result_Bus_Sig9 : ToWorkspace  VariableName=sig_result_009_009  SaveFormat=Structure With Time
  specifyOutputs : Subsystem
  result : Outport
  wires:
  sig_Req_Bus/1 -> BS/1, specifyOutputs/1(sig_Req_Bus)
  BS/1 -> ToWs_Req_Bus_Sig1/1  "<testSig_AccPed_trqDes>"
  BS/2 -> ToWs_Req_Bus_Sig2/1  "<testSig_APP_r>"
  BS/3 -> ToWs_Req_Bus_Sig3/1  "<testSig_CoETS_trqNTCActvOff>"
  BS/4 -> ToWs_Req_Bus_Sig4/1  "<testSig_CoETS_trqNTCActvOn>"
  BS/5 -> ToWs_Req_Bus_Sig5/1  "<testSig_CoETS_trqUnFltLtd>"
  BS/6 -> ToWs_Req_Bus_Sig6/1  "<testSig_CoVeh_trqAcs>"
  BS/7 -> ToWs_Req_Bus_Sig7/1  "<testSig_CoVeh_trqPrpLimErr>"
  BS/8 -> ToWs_Req_Bus_Sig8/1  "<testSig_CoVMD_trqLLim>"
  BS/9 -> ToWs_Req_Bus_Sig9/1  "<testSig_CrCtl_aAccThres>"
  BS/10 -> ToWs_Req_Bus_Sig10/1  "<testSig_CrCtl_aDeclThres>"
  BS/11 -> ToWs_Req_Bus_Sig11/1  "<testSig_CrCtl_st>"
  BS/12 -> ToWs_Req_Bus_Sig12/1  "<testSig_CrCtl_stGvnr>"
  BS/13 -> ToWs_Req_Bus_Sig13/1  "<testSig_CrCtl_stLck>"
  BS/14 -> ToWs_Req_Bus_Sig14/1  "<testSig_CrCtl_stShOff>"
  BS/15 -> ToWs_Req_Bus_Sig15/1  "<testSig_CrCtl_stSub>"
  BS/16 -> ToWs_Req_Bus_Sig16/1  "<testSig_CrCtl_stSubGvnr>"
  BS/17 -> ToWs_Req_Bus_Sig17/1  "<testSig_CrCtl_stSuspAct>"
  BS/18 -> ToWs_Req_Bus_Sig18/1  "<testSig_CrCtl_stVDirChng>"
  BS/19 -> ToWs_Req_Bus_Sig19/1  "<testSig_CrCtl_vDes>"
  BS/20 -> ToWs_Req_Bus_Sig20/1  "<testSig_CrCtl_vDesAct>"
  BS/21 -> ToWs_Req_Bus_Sig21/1  "<testSig_CrCtl_vDesActOld>"
  BS/22 -> ToWs_Req_Bus_Sig22/1  "<testSig_CrCtl_vMaxDvtAcc>"
  BS/23 -> ToWs_Req_Bus_Sig23/1  "<testSig_CrCtl_vMaxDvtDecl>"
  BS/24 -> ToWs_Req_Bus_Sig24/1  "<testSig_CrCtl_vMin>"
  BS/25 -> ToWs_Req_Bus_Sig25/1  "<testSig_EBrk_stPreSelMode>"
  BS/26 -> ToWs_Req_Bus_Sig26/1  "<testSig_EngDem_trqInrLim>"
  BS/27 -> ToWs_Req_Bus_Sig27/1  "<testSig_GlbDa_aXFlt>"
  BS/28 -> ToWs_Req_Bus_Sig28/1  "<testSig_GlbDa_vXFlt>"
  BS/29 -> ToWs_Req_Bus_Sig29/1  "<testSig_InjSys_trqLim>"
  BS/30 -> ToWs_Req_Bus_Sig30/1  "<testSig_PT_rTraV2N>"
  BS/31 -> ToWs_Req_Bus_Sig31/1  "<testSig_PT_rTrq>"
  BS/32 -> ToWs_Req_Bus_Sig32/1  "<testSig_PT_trqLos>"
  BS/33 -> ToWs_Req_Bus_Sig33/1  "<testSig_PT_trqWhl>"
  BS/34 -> ToWs_Req_Bus_Sig34/1  "<testSig_PT_trqWhlMinEng>"
  BS/35 -> ToWs_Req_Bus_Sig35/1  "<testSig_PT_trqWhlMinEngBrk>"
  BS/36 -> ToWs_Req_Bus_Sig36/1  "<testSig_RngMod_trqMin>"
  BS/37 -> ToWs_Req_Bus_Sig37/1  "<testSig_Tra_numGear>"
  BS/38 -> ToWs_Req_Bus_Sig38/1  "<testSig_VehMot_rTrqDfftl>"
  BS/39 -> ToWs_Req_Bus_Sig39/1  "<testSig_VMD_trqDes>"
  BS/40 -> ToWs_Req_Bus_Sig40/1  "<testSig_VMSAdjBtn_st>"
  BS/41 -> ToWs_Req_Bus_Sig41/1  "<testSig_VMSLmtSwt_st>"
  BS/42 -> ToWs_Req_Bus_Sig42/1  "<testSig_WESDem_stCurr>"
  BS/43 -> ToWs_Req_Bus_Sig43/1  "<testSig_CrCtl_rTraV2NBeg>"
  BS/44 -> ToWs_Req_Bus_Sig44/1  "<testSig_CrCtl_stOpFunc>"
  BS/45 -> ToWs_Req_Bus_Sig45/1  "<testSig_CrCtl_stPtd>"
  BS/46 -> ToWs_Req_Bus_Sig46/1  "<testSig_CrCtl_stReq>"
  BS/47 -> ToWs_Req_Bus_Sig47/1  "<testSig_CrCtl_stSuspRamp>"
  BS/48 -> ToWs_Req_Bus_Sig48/1  "<testSig_CrCtl_stvHysEngBrkReq>"
  BS/49 -> ToWs_Req_Bus_Sig49/1  "<testSig_CrCtl_trqLead>"
  BS/50 -> ToWs_Req_Bus_Sig50/1  "<testSig_CrCtl_trqLimAct>"
  BS/51 -> ToWs_Req_Bus_Sig51/1  "<testSig_CrCtl_trqMin>"
  BS/52 -> ToWs_Req_Bus_Sig52/1  "<testSig_CrCtl_trqReq>"
  BS/53 -> ToWs_Req_Bus_Sig53/1  "<testSig_CrCtl_trqReqOld>"
  BS/54 -> ToWs_Req_Bus_Sig54/1  "<testSig_CrCtl_vMax>"
  sig_Result_Bus/1 -> BS_Result/1, specifyOutputs/2(sig_Result_Bus)
  BS_Result/1 -> ToWs_Result_Bus_Sig1/1  "<CrCtl_rTraV2NBeg>"
  BS_Result/2 -> ToWs_Result_Bus_Sig2/1  "<CrCtl_stOpFunc>"
  BS_Result/3 -> ToWs_Result_Bus_Sig3/1  "<CrCtl_stPtd>"
  BS_Result/4 -> ToWs_Result_Bus_Sig4/1  "<CrCtl_stReq>"
  BS_Result/5 -> ToWs_Result_Bus_Sig5/1  "<CrCtl_stSuspRamp>"
  BS_Result/6 -> ToWs_Result_Bus_Sig6/1  "<CrCtl_stvHysEngBrkReq>"
  BS_Result/7 -> ToWs_Result_Bus_Sig7/1  "<CrCtl_trqLead>"
  BS_Result/8 -> ToWs_Result_Bus_Sig8/1  "<CrCtl_trqLimAct>"
  BS_Result/9 -> ToWs_Result_Bus_Sig9/1  "<CrCtl_trqMin>"
  BS_Result/10 -> ToWs_Result_Bus_Sig10/1  "<CrCtl_trqReq>"
  BS_Result/11 -> ToWs_Result_Bus_Sig11/1  "<CrCtl_trqReqOld>"
  BS_Result/12 -> ToWs_Result_Bus_Sig12/1  "<CrCtl_vMax>"
  specifyOutputs/1(result) -> result/1

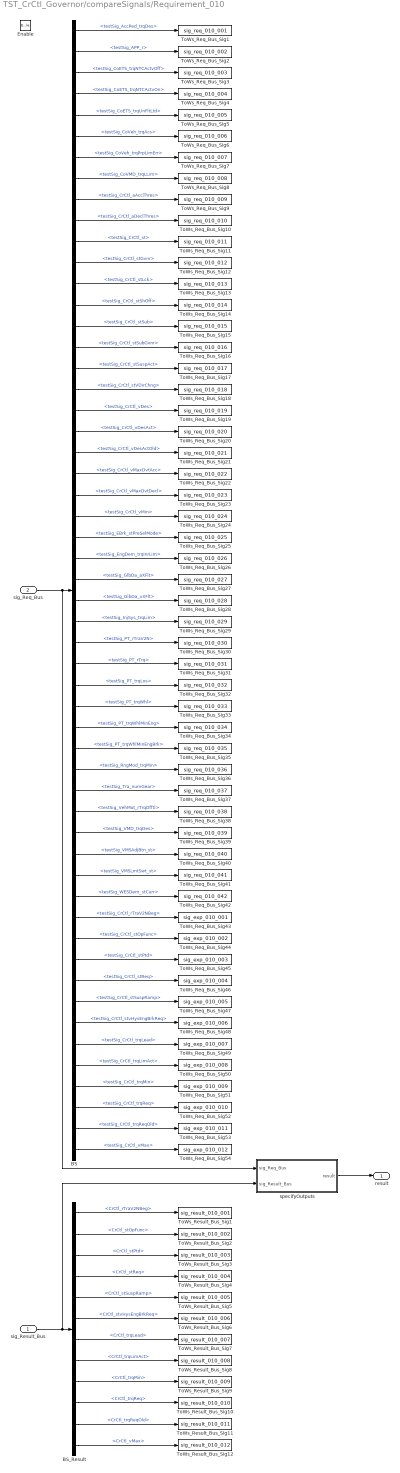
== system TST_CrCtl_Governor/compareSignals/Requirement_010 ==
  sig_Result_Bus : Inport
  sig_Req_Bus : Inport  Port=2
  Enable : EnablePort
  BS : BusSelector  OutputSignals=testSig_AccPed_trqDes,testSig_APP_r,testSig_CoETS_trqNTCActvOff,testSig_CoETS_trqNTCActvOn,testSig_CoETS_trqUnFltLtd,testSig_CoVeh_trqAcs,testSig_CoVeh_trqPrpLimErr,testSig_CoVMD_trqLLim,testSig_CrCtl_aAccThres,testSig_CrCtl_aDeclThres,testSig_CrCtl_st,testSig_CrCtl_stGvnr,testSig_CrCtl_stLck,testSig_CrCtl_stShOff,testSig_CrCtl_stSub,testSig_CrCtl_stSubGvnr,testSig_CrCtl_stSuspAct,testSig_CrCtl_stVDirChng,testSig_CrCtl_vDes,testSig_CrCtl_vDesAct,testSig_CrCtl_vDesActOld,testSig_CrCtl_vMaxDvtAcc,testSig_CrCtl_vMaxDvtDecl,testSig_CrCtl_vMin,testSig_EBrk_stPreSelMode,testSig_EngDem_trqInrLim,testSig_GlbDa_aXFlt,testSig_GlbDa_vXFlt,testSig_InjSys_trqLim,testSig_PT_rTraV2N,testSig_PT_rTrq,testSig_PT_trqLos,testSig_PT_trqWhl,testSig_PT_trqWhlMinEng,testSig_PT_trqWhlMinEngBrk,testSig_RngMod_trqMin,testSig_Tra_numGear,testSig_VehMot_rTrqDfftl,testSig_VMD_trqDes,testSig_VMSAdjBtn_st,testSig_VMSLmtSwt_st,testSig_WESDem_stCurr,testSig_CrCtl_rTraV2NBeg,testSig_CrCtl_stOpFunc,testSig_CrCtl_stPtd,testSig_CrCtl_stReq,testSig_CrCtl_stSuspRamp,testSig_CrCtl_stvHysEngBrkReq,testSig_CrCtl_trqLead,testSig_CrCtl_trqLimAct,testSig_CrCtl_trqMin,testSig_CrCtl_trqReq,testSig_CrCtl_trqReqOld,testSig_CrCtl_vMax
  BS_Result : BusSelector  OutputSignals=CrCtl_rTraV2NBeg,CrCtl_stOpFunc,CrCtl_stPtd,CrCtl_stReq,CrCtl_stSuspRamp,CrCtl_stvHysEngBrkReq,CrCtl_trqLead,CrCtl_trqLimAct,CrCtl_trqMin,CrCtl_trqReq,CrCtl_trqReqOld,CrCtl_vMax
  ToWs_Req_Bus_Sig1 : ToWorkspace  VariableName=sig_req_010_001  SaveFormat=Structure With Time
  ToWs_Req_Bus_Sig10 : ToWorkspace  VariableName=sig_req_010_010  SaveFormat=Structure With Time
  ToWs_Req_Bus_Sig11 : ToWorkspace  VariableName=sig_req_010_011  SaveFormat=Structure With Time
  ToWs_Req_Bus_Sig12 : ToWorkspace  VariableName=sig_req_010_012  SaveFormat=Structure With Time
  ToWs_Req_Bus_Sig13 : ToWorkspace  VariableName=sig_req_010_013  SaveFormat=Structure With Time
  ToWs_Req_Bus_Sig14 : ToWorkspace  VariableName=sig_req_010_014  SaveFormat=Structure With Time
  ToWs_Req_Bus_Sig15 : ToWorkspace  VariableName=sig_req_010_015  SaveFormat=Structure With Time
  ToWs_Req_Bus_Sig16 : ToWorkspace  VariableName=sig_req_010_016  SaveFormat=Structure With Time
  ToWs_Req_Bus_Sig17 : ToWorkspace  VariableName=sig_req_010_017  SaveFormat=Structure With Time
  ToWs_Req_Bus_Sig18 : ToWorkspace  VariableName=sig_req_010_018  SaveFormat=Structure With Time
  ToWs_Req_Bus_Sig19 : ToWorkspace  VariableName=sig_req_010_019  SaveFormat=Structure With Time
  ToWs_Req_Bus_Sig2 : ToWorkspace  VariableName=sig_req_010_002  SaveFormat=Structure With Time
  ToWs_Req_Bus_Sig20 : ToWorkspace  VariableName=sig_req_010_020  SaveFormat=Structure With Time
  ToWs_Req_Bus_Sig21 : ToWorkspace  VariableName=sig_req_010_021  SaveFormat=Structure With Time
  ToWs_Req_Bus_Sig22 : ToWorkspace  VariableName=sig_req_010_022  SaveFormat=Structure With Time
  ToWs_Req_Bus_Sig23 : ToWorkspace  VariableName=sig_req_010_023  SaveFormat=Structure With Time
  ToWs_Req_Bus_Sig24 : ToWorkspace  VariableName=sig_req_010_024  SaveFormat=Structure With Time
  ToWs_Req_Bus_Sig25 : ToWorkspace  VariableName=sig_req_010_025  SaveFormat=Structure With Time
  ToWs_Req_Bus_Sig26 : ToWorkspace  VariableName=sig_req_010_026  SaveFormat=Structure With Time
  ToWs_Req_Bus_Sig27 : ToWorkspace  VariableName=sig_req_010_027  SaveFormat=Structure With Time
  ToWs_Req_Bus_Sig28 : ToWorkspace  VariableName=sig_req_010_028  SaveFormat=Structure With Time
  ToWs_Req_Bus_Sig29 : ToWorkspace  VariableName=sig_req_010_029  SaveFormat=Structure With Time
  ToWs_Req_Bus_Sig3 : ToWorkspace  VariableName=sig_req_010_003  SaveFormat=Structure With Time
  ToWs_Req_Bus_Sig30 : ToWorkspace  VariableName=sig_req_010_030  SaveFormat=Structure With Time
  ToWs_Req_Bus_Sig31 : ToWorkspace  VariableName=sig_req_010_031  SaveFormat=Structure With Time
  ToWs_Req_Bus_Sig32 : ToWorkspace  VariableName=sig_req_010_032  SaveFormat=Structure With Time
  ToWs_Req_Bus_Sig33 : ToWorkspace  VariableName=sig_req_010_033  SaveFormat=Structure With Time
  ToWs_Req_Bus_Sig34 : ToWorkspace  VariableName=sig_req_010_034  SaveFormat=Structure With Time
  ToWs_Req_Bus_Sig35 : ToWorkspace  VariableName=sig_req_010_035  SaveFormat=Structure With Time
  ToWs_Req_Bus_Sig36 : ToWorkspace  VariableName=sig_req_010_036  SaveFormat=Structure With Time
  ToWs_Req_Bus_Sig37 : ToWorkspace  VariableName=sig_req_010_037  SaveFormat=Structure With Time
  ToWs_Req_Bus_Sig38 : ToWorkspace  VariableName=sig_req_010_038  SaveFormat=Structure With Time
  ToWs_Req_Bus_Sig39 : ToWorkspace  VariableName=sig_req_010_039  SaveFormat=Structure With Time
  ToWs_Req_Bus_Sig4 : ToWorkspace  VariableName=sig_req_010_004  SaveFormat=Structure With Time
  ToWs_Req_Bus_Sig40 : ToWorkspace  VariableName=sig_req_010_040  SaveFormat=Structure With Time
  ToWs_Req_Bus_Sig41 : ToWorkspace  VariableName=sig_req_010_041  SaveFormat=Structure With Time
  ToWs_Req_Bus_Sig42 : ToWorkspace  VariableName=sig_req_010_042  SaveFormat=Structure With Time
  ToWs_Req_Bus_Sig43 : ToWorkspace  VariableName=sig_exp_010_001  SaveFormat=Structure With Time
  ToWs_Req_Bus_Sig44 : ToWorkspace  VariableName=sig_exp_010_002  SaveFormat=Structure With Time
  ToWs_Req_Bus_Sig45 : ToWorkspace  VariableName=sig_exp_010_003  SaveFormat=Structure With Time
  ToWs_Req_Bus_Sig46 : ToWorkspace  VariableName=sig_exp_010_004  SaveFormat=Structure With Time
  ToWs_Req_Bus_Sig47 : ToWorkspace  VariableName=sig_exp_010_005  SaveFormat=Structure With Time
  ToWs_Req_Bus_Sig48 : ToWorkspace  VariableName=sig_exp_010_006  SaveFormat=Structure With Time
  ToWs_Req_Bus_Sig49 : ToWorkspace  VariableName=sig_exp_010_007  SaveFormat=Structure With Time
  ToWs_Req_Bus_Sig5 : ToWorkspace  VariableName=sig_req_010_005  SaveFormat=Structure With Time
  ToWs_Req_Bus_Sig50 : ToWorkspace  VariableName=sig_exp_010_008  SaveFormat=Structure With Time
  ToWs_Req_Bus_Sig51 : ToWorkspace  VariableName=sig_exp_010_009  SaveFormat=Structure With Time
  ToWs_Req_Bus_Sig52 : ToWorkspace  VariableName=sig_exp_010_010  SaveFormat=Structure With Time
  ToWs_Req_Bus_Sig53 : ToWorkspace  VariableName=sig_exp_010_011  SaveFormat=Structure With Time
  ToWs_Req_Bus_Sig54 : ToWorkspace  VariableName=sig_exp_010_012  SaveFormat=Structure With Time
  ToWs_Req_Bus_Sig6 : ToWorkspace  VariableName=sig_req_010_006  SaveFormat=Structure With Time
  ToWs_Req_Bus_Sig7 : ToWorkspace  VariableName=sig_req_010_007  SaveFormat=Structure With Time
  ToWs_Req_Bus_Sig8 : ToWorkspace  VariableName=sig_req_010_008  SaveFormat=Structure With Time
  ToWs_Req_Bus_Sig9 : ToWorkspace  VariableName=sig_req_010_009  SaveFormat=Structure With Time
  ToWs_Result_Bus_Sig1 : ToWorkspace  VariableName=sig_result_010_001  SaveFormat=Structure With Time
  ToWs_Result_Bus_Sig10 : ToWorkspace  VariableName=sig_result_010_010  SaveFormat=Structure With Time
  ToWs_Result_Bus_Sig11 : ToWorkspace  VariableName=sig_result_010_011  SaveFormat=Structure With Time
  ToWs_Result_Bus_Sig12 : ToWorkspace  VariableName=sig_result_010_012  SaveFormat=Structure With Time
  ToWs_Result_Bus_Sig2 : ToWorkspace  VariableName=sig_result_010_002  SaveFormat=Structure With Time
  ToWs_Result_Bus_Sig3 : ToWorkspace  VariableName=sig_result_010_003  SaveFormat=Structure With Time
  ToWs_Result_Bus_Sig4 : ToWorkspace  VariableName=sig_result_010_004  SaveFormat=Structure With Time
  ToWs_Result_Bus_Sig5 : ToWorkspace  VariableName=sig_result_010_005  SaveFormat=Structure With Time
  ToWs_Result_Bus_Sig6 : ToWorkspace  VariableName=sig_result_010_006  SaveFormat=Structure With Time
  ToWs_Result_Bus_Sig7 : ToWorkspace  VariableName=sig_result_010_007  SaveFormat=Structure With Time
  ToWs_Result_Bus_Sig8 : ToWorkspace  VariableName=sig_result_010_008  SaveFormat=Structure With Time
  ToWs_Result_Bus_Sig9 : ToWorkspace  VariableName=sig_result_010_009  SaveFormat=Structure With Time
  specifyOutputs : Subsystem
  result : Outport
  wires:
  sig_Req_Bus/1 -> BS/1, specifyOutputs/1(sig_Req_Bus)
  BS/1 -> ToWs_Req_Bus_Sig1/1  "<testSig_AccPed_trqDes>"
  BS/2 -> ToWs_Req_Bus_Sig2/1  "<testSig_APP_r>"
  BS/3 -> ToWs_Req_Bus_Sig3/1  "<testSig_CoETS_trqNTCActvOff>"
  BS/4 -> ToWs_Req_Bus_Sig4/1  "<testSig_CoETS_trqNTCActvOn>"
  BS/5 -> ToWs_Req_Bus_Sig5/1  "<testSig_CoETS_trqUnFltLtd>"
  BS/6 -> ToWs_Req_Bus_Sig6/1  "<testSig_CoVeh_trqAcs>"
  BS/7 -> ToWs_Req_Bus_Sig7/1  "<testSig_CoVeh_trqPrpLimErr>"
  BS/8 -> ToWs_Req_Bus_Sig8/1  "<testSig_CoVMD_trqLLim>"
  BS/9 -> ToWs_Req_Bus_Sig9/1  "<testSig_CrCtl_aAccThres>"
  BS/10 -> ToWs_Req_Bus_Sig10/1  "<testSig_CrCtl_aDeclThres>"
  BS/11 -> ToWs_Req_Bus_Sig11/1  "<testSig_CrCtl_st>"
  BS/12 -> ToWs_Req_Bus_Sig12/1  "<testSig_CrCtl_stGvnr>"
  BS/13 -> ToWs_Req_Bus_Sig13/1  "<testSig_CrCtl_stLck>"
  BS/14 -> ToWs_Req_Bus_Sig14/1  "<testSig_CrCtl_stShOff>"
  BS/15 -> ToWs_Req_Bus_Sig15/1  "<testSig_CrCtl_stSub>"
  BS/16 -> ToWs_Req_Bus_Sig16/1  "<testSig_CrCtl_stSubGvnr>"
  BS/17 -> ToWs_Req_Bus_Sig17/1  "<testSig_CrCtl_stSuspAct>"
  BS/18 -> ToWs_Req_Bus_Sig18/1  "<testSig_CrCtl_stVDirChng>"
  BS/19 -> ToWs_Req_Bus_Sig19/1  "<testSig_CrCtl_vDes>"
  BS/20 -> ToWs_Req_Bus_Sig20/1  "<testSig_CrCtl_vDesAct>"
  BS/21 -> ToWs_Req_Bus_Sig21/1  "<testSig_CrCtl_vDesActOld>"
  BS/22 -> ToWs_Req_Bus_Sig22/1  "<testSig_CrCtl_vMaxDvtAcc>"
  BS/23 -> ToWs_Req_Bus_Sig23/1  "<testSig_CrCtl_vMaxDvtDecl>"
  BS/24 -> ToWs_Req_Bus_Sig24/1  "<testSig_CrCtl_vMin>"
  BS/25 -> ToWs_Req_Bus_Sig25/1  "<testSig_EBrk_stPreSelMode>"
  BS/26 -> ToWs_Req_Bus_Sig26/1  "<testSig_EngDem_trqInrLim>"
  BS/27 -> ToWs_Req_Bus_Sig27/1  "<testSig_GlbDa_aXFlt>"
  BS/28 -> ToWs_Req_Bus_Sig28/1  "<testSig_GlbDa_vXFlt>"
  BS/29 -> ToWs_Req_Bus_Sig29/1  "<testSig_InjSys_trqLim>"
  BS/30 -> ToWs_Req_Bus_Sig30/1  "<testSig_PT_rTraV2N>"
  BS/31 -> ToWs_Req_Bus_Sig31/1  "<testSig_PT_rTrq>"
  BS/32 -> ToWs_Req_Bus_Sig32/1  "<testSig_PT_trqLos>"
  BS/33 -> ToWs_Req_Bus_Sig33/1  "<testSig_PT_trqWhl>"
  BS/34 -> ToWs_Req_Bus_Sig34/1  "<testSig_PT_trqWhlMinEng>"
  BS/35 -> ToWs_Req_Bus_Sig35/1  "<testSig_PT_trqWhlMinEngBrk>"
  BS/36 -> ToWs_Req_Bus_Sig36/1  "<testSig_RngMod_trqMin>"
  BS/37 -> ToWs_Req_Bus_Sig37/1  "<testSig_Tra_numGear>"
  BS/38 -> ToWs_Req_Bus_Sig38/1  "<testSig_VehMot_rTrqDfftl>"
  BS/39 -> ToWs_Req_Bus_Sig39/1  "<testSig_VMD_trqDes>"
  BS/40 -> ToWs_Req_Bus_Sig40/1  "<testSig_VMSAdjBtn_st>"
  BS/41 -> ToWs_Req_Bus_Sig41/1  "<testSig_VMSLmtSwt_st>"
  BS/42 -> ToWs_Req_Bus_Sig42/1  "<testSig_WESDem_stCurr>"
  BS/43 -> ToWs_Req_Bus_Sig43/1  "<testSig_CrCtl_rTraV2NBeg>"
  BS/44 -> ToWs_Req_Bus_Sig44/1  "<testSig_CrCtl_stOpFunc>"
  BS/45 -> ToWs_Req_Bus_Sig45/1  "<testSig_CrCtl_stPtd>"
  BS/46 -> ToWs_Req_Bus_Sig46/1  "<testSig_CrCtl_stReq>"
  BS/47 -> ToWs_Req_Bus_Sig47/1  "<testSig_CrCtl_stSuspRamp>"
  BS/48 -> ToWs_Req_Bus_Sig48/1  "<testSig_CrCtl_stvHysEngBrkReq>"
  BS/49 -> ToWs_Req_Bus_Sig49/1  "<testSig_CrCtl_trqLead>"
  BS/50 -> ToWs_Req_Bus_Sig50/1  "<testSig_CrCtl_trqLimAct>"
  BS/51 -> ToWs_Req_Bus_Sig51/1  "<testSig_CrCtl_trqMin>"
  BS/52 -> ToWs_Req_Bus_Sig52/1  "<testSig_CrCtl_trqReq>"
  BS/53 -> ToWs_Req_Bus_Sig53/1  "<testSig_CrCtl_trqReqOld>"
  BS/54 -> ToWs_Req_Bus_Sig54/1  "<testSig_CrCtl_vMax>"
  sig_Result_Bus/1 -> BS_Result/1, specifyOutputs/2(sig_Result_Bus)
  BS_Result/1 -> ToWs_Result_Bus_Sig1/1  "<CrCtl_rTraV2NBeg>"
  BS_Result/2 -> ToWs_Result_Bus_Sig2/1  "<CrCtl_stOpFunc>"
  BS_Result/3 -> ToWs_Result_Bus_Sig3/1  "<CrCtl_stPtd>"
  BS_Result/4 -> ToWs_Result_Bus_Sig4/1  "<CrCtl_stReq>"
  BS_Result/5 -> ToWs_Result_Bus_Sig5/1  "<CrCtl_stSuspRamp>"
  BS_Result/6 -> ToWs_Result_Bus_Sig6/1  "<CrCtl_stvHysEngBrkReq>"
  BS_Result/7 -> ToWs_Result_Bus_Sig7/1  "<CrCtl_trqLead>"
  BS_Result/8 -> ToWs_Result_Bus_Sig8/1  "<CrCtl_trqLimAct>"
  BS_Result/9 -> ToWs_Result_Bus_Sig9/1  "<CrCtl_trqMin>"
  BS_Result/10 -> ToWs_Result_Bus_Sig10/1  "<CrCtl_trqReq>"
  BS_Result/11 -> ToWs_Result_Bus_Sig11/1  "<CrCtl_trqReqOld>"
  BS_Result/12 -> ToWs_Result_Bus_Sig12/1  "<CrCtl_vMax>"
  specifyOutputs/1(result) -> result/1
